simulink model "HW2_Theory_task5"  (R2023b)
settings: Solver=VariableStepAuto  StartTime=0.0  StopTime=10.0  RelTol=1e-3
settings Model: Creator=Admin  LastModifiedBy=Admin

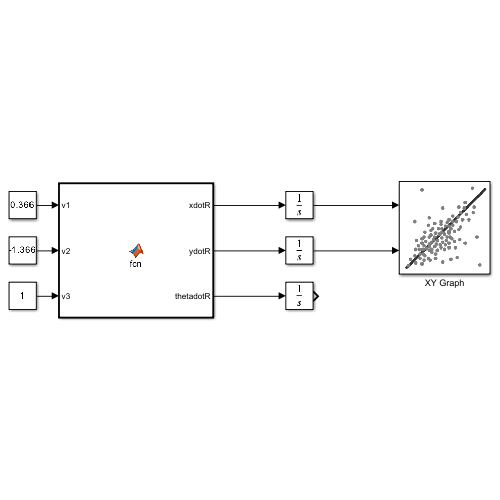
[thumbnail: Simulink's stored preview of the top-level diagram]
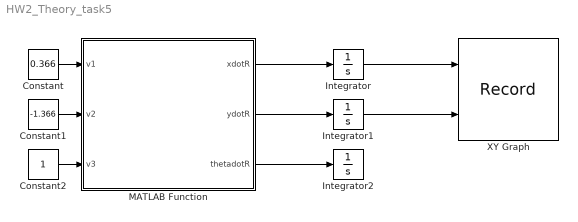
== system HW2_Theory_task5 ==
  Constant : Constant  Value=0.366
  Constant1 : Constant  Value=-1.366
  Constant2 : Constant
  Integrator : Integrator
  Integrator1 : Integrator
  Integrator2 : Integrator
  MATLAB Function : MATLAB Function  TreatAsAtomicUnit=on
  XY Graph : Record  FileSettingsInternal="{\"entries\":[{\"content\":{\"excelSettings\":{\"content\":{},\"type\":\"Streamout.ExcelSettings\"}},\"type\":\"Streamout.FileSettingStorage\",\"uuid\":\"\"}],\"packageUris\":[\"http:\\/\\/schema.mathworks.com\\/mf0\\/streamout_blocks\\/R2020a\"],\"version\":\"1.0\"}"  Layout=[1 1]  SignalsInternal="{\"entries\":[{\"content\":{\"signals\":[{\"content\":{\"blockPath\":[],\"dimensions\":[1],\"domain\":\"\",\"lineColor\":\"#a2142f\",\"plots\":[1],\"port\":1,\"sid\":[\"\"],\"signalID\":168,\"signalName\":\"Integrator\"},\"type\":\"RecordBlkView.Signal\",\"uuid\":\"\"},{\"content\":{\"blockPath\":[],\"dimensions\":[1],\"domain\":\"\",\"lineColor\":\"#139fff\",\"plots\":[1],\"port\":2,\"sid\":[\"\"],\"signalID\":172,\"signalName\":\"Integrator1\"},\"type\":\"RecordBlkView.Signal\",\"uuid\":\"\"}]},\"type\":\"RecordBlkView.InputSignals\",\"uuid\":\"\"}],\"packageUris\":[\"http:\\/\\/schema.mathworks.com\\/mf0\\/streamout_blocks\\/R2020a\"],\"version\":\"1.0\"}"  VisualizationBindings="{\"xyplotplugin\":{\"info\":[{\"series\":[{\"bindingParametersList\":[{\"parameter\":\"X-Axis\",\"signalID\":168,\"signalName\":\"Integrator\"},{\"parameter\":\"Y-Axis\",\"signalID\":172,\"signalName\":\"Integrator1\"}],\"seriesID\":54715}],\"subplotID\":1}]}}"  CompatibilityTag=XY
  wires:
  MATLAB Function/2(ydotR) -> Integrator1/1
  MATLAB Function/1(xdotR) -> Integrator/1
  MATLAB Function/3(thetadotR) -> Integrator2/1
  Constant/1 -> MATLAB Function/1(v1)
  Constant1/1 -> MATLAB Function/2(v2)
  Constant2/1 -> MATLAB Function/3(v3)
  Integrator/1 -> XY Graph/1
  Integrator1/1 -> XY Graph/2

== matlab function HW2_Theory_task5/MATLAB Function ==
  data: v1 input; xdotR output; v2 input; v3 input; ydotR output; thetadotR output
function [xdotR, ydotR, thetadotR]= fcn(v1,v2,v3)
l = 1;
xdotR = [1/sqrt(3) -1/sqrt(3) 0] * [v1;v2;v3];
ydotR = [-1/3 -1/3 2/3] * [v1;v2;v3];
thetadotR = [-1/(3*l) -1/(3*l) -1/(3*l)] * [v1;v2;v3];
